simulink model "LDSNEmo_TestBench"  (R2020b)
settings: Solver=FixedStepAuto  StartTime=0.0  StopTime=1477  FixedStep=0.01  RelTol=1e-3
model workspace (MAT data in the model file):
  C_RR = 0.0103752252297
  SampleTime = 0.01
  StopTime = 1477
  UncertaintyRollerDynamometer = 0.796984855506
  VehMass = 929
  c_w = 0.37
  cycle : timeseries (value not decoded)
  i_gear = 5.6813
  p = 2.5
  power_map_LE = [81.3594367777 81.3594367777 88.9151238368 69.3920543425 121.856227925 33.5913037104 56.5214963128 60.6342218487 61.1595876762 53.4292335319 53.4133899816 35.6771556802 ... (16260 elements, 60x271)]
  power_map_Mot = [0 74.834999341 40.2428359465 95.3690451807 75.6091573236 114.707467852 143.074401876 144.922747771 177.284289075 184.351766643 192.404587732 197.413952644 ... (16260 elements, 60x271)]
  r_dyn = 0.275233869952
undefined symbols (not defined in the file): DiscIntNeverNeededParam, gravity, UncertaintyMappedLosses, UncertaintyTabledConsumption, v_HA
libraries: Constant_Environment x1, Driver_PI x1, Longitudinal_DrivingCycles x1, Acceleration_Calculation x1, Air_Resistance x1, Roll_Resistance x1, Slope_Resistance x1, Simple_Auxiliary x1, Electric_Drive_Tabled_Consumption x1, Gear_Stage x1, DCAC_Converter x1, Control_Unit_Simple x1
(part 2 of 3)

== system LDSNEmo_TestBench/Driver and Environment ==
  BUS_In : Inport
  BUS IN : Subsystem
      mask help:
      | <Author> Alexander Koch based on Stefan Müller, Stephan Rohr
      | <Date> 02/05/2017
      |
      | <Description>
      | Automated BUS IN Block for the Bus System. After the Bus In is connected and receives signals it is possible to choose the required signals by clicking on the block. After choosing the signals it is possible to push the Refresh button. This button builds the required amount of outputs, connects the Bus Selector and the Outputs and rename all the outputs with the corresponding signal name.
      |
      | The Block automaticlly disconnects the link to the library block after opening the first time
      |
      | <Parameters>
      | -
      |
      | <Inputs>
      | Bus [Bus]
      |
      | <Outputs>
      | Bus [Bus]
      | SignalName[-]
      mask init:
      | BusInInitFct()
      settings: OpenFcn=|
      | set_param(gcb(),'LinkStatus','none')
      | open_system(gcb(),'mask')
      | open_system(strcat(gcb(),'/Bus Selector'),'Parameter')
      mask DialogControl ParameterGroupVar Prompt: Refresh
      mask DialogControl RefreshOutputs Prompt: Refresh all Output Names
      mask DialogControl RefreshOutputs Callback: BusInInitFct()
  BUS OUT : Subsystem  mask{NumberofInputs=6, NameSys='Driver and Enironment'}
      mask prompts: NumberofInputs "Numper of costum inputs"; NameSys "Name of Bus Subsystem"
      mask help:
      | <Author> Alexander Koch based on Stefan Müller, Stephan Rohr
      | <Date> 02/05/2017
      |
      | <Description>
      | Automated BUS Out Block for the Bus System. Allows to enter the Number of costum inputs and the name of the bus system. After entering the parameters the required amout of Inputs are built and connected to the Bus Creator. The signal names that are connected to the inputs In1, ..., InN are automatically adopted at the Bus signal names and can be found in the Bus under the name of the Bus Subsystem. If the signal (line) to the Inport has no name, the name of the previous blocks outport is taken. If this is not possible, the name if the previous block is taken for the Bus signal name.
      |
      | Additional, there are two buttons. The Refresh Input Names refreshes all Input Names. This is required if signal names are changed or signals are connected for the first time. To build a new system or if another Subsystem is added between existing subsystems, the Refresh Bus Selector is required at every subsystem that is calculated after the new subsystem.
      |
      | The Block automaticlly disconnects the link to the library block after opening the first time
      |
      | <Parameters>
      | Number of costum inputs [-]
      | Name of Bus Subsystem ['abc']
      |
      | <Inputs>
      | Bus [Bus]
      | In1 [ ]
      |
      | <Outputs>
      | Bus [Bus]
      mask init:
      | BusRefreshInputs()
      settings: OpenFcn=|
      | set_param(gcb(),'LinkStatus','none')
      | open_system(gcb(),'mask')
      mask DialogControl Container3 Prompt: Refresh
      mask DialogControl RefreshInputNames Prompt: Refresh Input Names
      mask DialogControl RefreshInputNames Callback: BusRefreshLineNames()
      mask DialogControl RefreshBusSelector Prompt: Refresh Bus Selector
      mask DialogControl RefreshBusSelector Callback: BusRefreshBusSelector()
  Constant Environment : Constant_Environment/Constant Environment  Ground_Slope=0  Long_Wind_Speed=0  Ambient_P=101325  Ambient_Temp=293.15  LocalSampleTime=-1
  Driver PI : Driver_PI/Driver PI  ThrottleP=7  ThrottleI=1  BrakeP=7  BrakeI=1.5  WeightingFactorPrecontrol=0  MaxVehicleSpeed=80  hysteresis=0.05  LocalSampleTime=-1
  BUS_Out : Outport  VectorParamsAs1DForOutWhenUnconnected=off
  wires:
  BUS IN/1(BUS) -> BUS OUT/1(BUS)
  BUS OUT/1(BUS_OUT) -> BUS_Out/1
  BUS_In/1 -> BUS IN/1(BUS_In)
  BUS IN/2(v [m/s]) -> Driver PI/1
  Driver PI/1 -> BUS OUT/2(In1)
  Driver PI/2 -> BUS OUT/3(In2)
  Constant Environment/1 -> BUS OUT/4(In3)
  Constant Environment/2 -> BUS OUT/5(In4)
  BUS IN/3(VehSpd [m/s]) -> Driver PI/2
  Constant Environment/3 -> BUS OUT/6(In5)
  Constant Environment/4 -> BUS OUT/7(In6)

== system LDSNEmo_TestBench/Driving Cycle ==
  BUS_In : Inport
  BUS IN : Subsystem
      mask help:
      | <Author> Alexander Koch
      | <Date> 02/05/2017
      | <Predecessor> Stefan Müller, Stephan Rohr
      |
      | <Description>
      | Automated BUS IN Block for the Bus System. After the Bus In is connected and receives signals it is possible to choose the required signals by clicking on the block. After choosing the signals it is possible to push the Refresh button. This button builds the required amount of outputs, connects the Bus Selector and the Outputs and rename all the outputs with the corresponding signal name.
      |
      | The Block automaticlly disconnects the link to the library block after opening the first time
      |
      | <Parameters>
      | -
      |
      | <Inputs>
      | Bus [Bus]
      |
      | <Outputs>
      | Bus [Bus]
      | SignalName[-]
      mask init:
      | BusInInitFct()
      settings: OpenFcn=|
      | set_param(gcb(),'LinkStatus','none')
      | open_system(gcb(),'mask')
      | open_system(strcat(gcb(),'/Bus Selector'),'Parameter')
      mask DialogControl ParameterGroupVar Prompt: Refresh
      mask DialogControl RefreshOutputs Prompt: Refresh all Output Names
      mask DialogControl RefreshOutputs Callback: BusInInitFct()
  BUS OUT : Subsystem  mask{NumberofInputs=4, NameSys='DrivinCycle'}
      mask prompts: NumberofInputs "Numper of costum inputs"; NameSys "Name of Bus Subsystem"
      mask help:
      | <Author> Alexander Koch based on Stefan Müller, Stephan Rohr
      | <Date> 02/05/2017
      |
      | <Description>
      | Automated BUS Out Block for the Bus System. Allows to enter the Number of costum inputs and the name of the bus system. After entering the parameters the required amout of Inputs are built and connected to the Bus Creator. The signal names that are connected to the inputs In1, ..., InN are automatically adopted at the Bus signal names and can be found in the Bus under the name of the Bus Subsystem. If the signal (line) to the Inport has no name, the name of the previous blocks outport is taken. If this is not possible, the name if the previous block is taken for the Bus signal name.
      |
      | Additional, there are two buttons. The Refresh Input Names refreshes all Input Names. This is required if signal names are changed or signals are connected for the first time. To build a new system or if another Subsystem is added between existing subsystems, the Refresh Bus Selector is required at every subsystem that is calculated after the new subsystem.
      |
      | The Block automaticlly disconnects the link to the library block after opening the first time
      |
      | <Parameters>
      | Number of costum inputs [-]
      | Name of Bus Subsystem ['abc']
      |
      | <Inputs>
      | Bus [Bus]
      | In1 [ ]
      |
      | <Outputs>
      | Bus [Bus]
      mask init:
      | BusRefreshInputs()
      settings: OpenFcn=|
      | set_param(gcb(),'LinkStatus','none')
      | open_system(gcb(),'mask')
      mask DialogControl Container3 Prompt: Refresh
      mask DialogControl RefreshInputNames Prompt: Refresh Input Names
      mask DialogControl RefreshInputNames Callback: BusRefreshLineNames()
      mask DialogControl RefreshBusSelector Prompt: Refresh Bus Selector
      mask DialogControl RefreshBusSelector Callback: BusRefreshBusSelector()
  Longitudinal Driving Cycles : Longitudinal_DrivingCycles/Longitudinal Driving Cycles  dcname=Custom_Driving_Cycle  dccircuits=1  dc_speed=cycle  dc_gear=[]  LocalSampleTime=-1
  Terminator : Terminator
  BUS_Out : Outport  VectorParamsAs1DForOutWhenUnconnected=off
  wires:
  BUS IN/1(BUS) -> BUS OUT/1(BUS)
  BUS OUT/1(BUS_OUT) -> BUS_Out/1
  BUS_In/1 -> BUS IN/1(BUS_In)
  Longitudinal Driving Cycles/1 -> BUS OUT/2(In1)  "v [m/s]"
  Longitudinal Driving Cycles/2 -> BUS OUT/3(In2)
  Longitudinal Driving Cycles/3 -> BUS OUT/4(In3)
  Longitudinal Driving Cycles/4 -> BUS OUT/5(In4)
  BUS IN/2(VehSpd [m/s]) -> Terminator/1

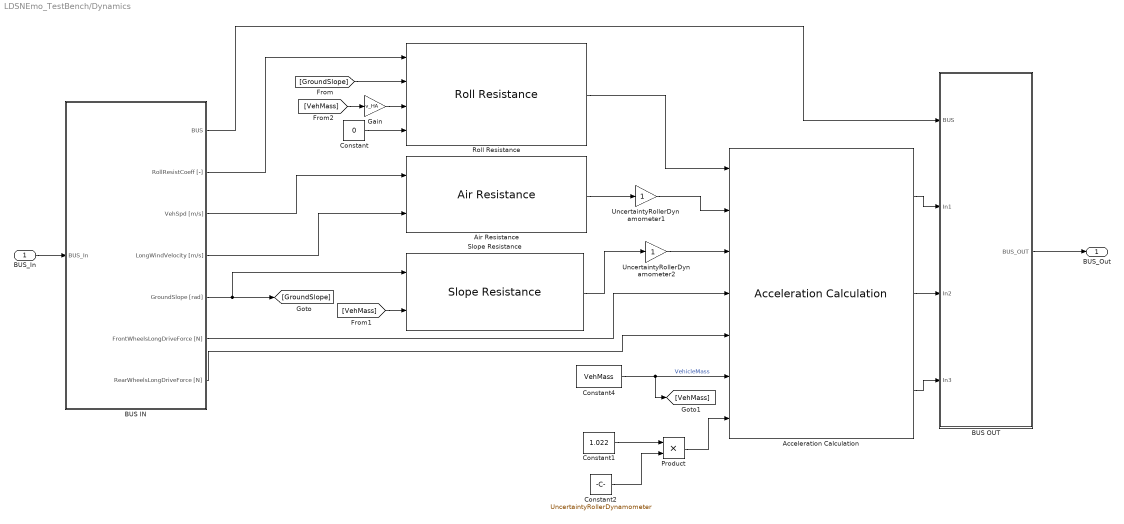
== system LDSNEmo_TestBench/Dynamics ==
  BUS_In : Inport
  Acceleration Calculation : Acceleration_Calculation/Acceleration Calculation  InitialCondition=0  LocalSampleTime=-1
  Air Resistance : Air_Resistance/Air Resistance  A_st=1.96  Roh_Air=rho_L  c_w=c_w  LocalSampleTime=-1
  BUS IN : Subsystem
      mask help:
      | <Author> Alexander Koch
      | <Date> 02/05/2017
      | <Predecessor> Stefan Müller, Stephan Rohr
      |
      | <Description>
      | Automated BUS IN Block for the Bus System. After the Bus In is connected and receives signals it is possible to choose the required signals by clicking on the block. After choosing the signals it is possible to push the Refresh button. This button builds the required amount of outputs, connects the Bus Selector and the Outputs and rename all the outputs with the corresponding signal name.
      |
      | The Block automaticlly disconnects the link to the library block after opening the first time
      |
      | <Parameters>
      | -
      |
      | <Inputs>
      | Bus [Bus]
      |
      | <Outputs>
      | Bus [Bus]
      | SignalName[-]
      mask init:
      | BusInInitFct()
      settings: OpenFcn=|
      | set_param(gcb(),'LinkStatus','none')
      | open_system(gcb(),'mask')
      | open_system(strcat(gcb(),'/Bus Selector'),'Parameter')
      mask DialogControl ParameterGroupVar Prompt: Refresh
      mask DialogControl RefreshOutputs Prompt: Refresh all Output Names
      mask DialogControl RefreshOutputs Callback: BusInInitFct()
  BUS OUT : Subsystem  mask{NumberofInputs=3, NameSys='Dynamics'}
      mask prompts: NumberofInputs "Numper of costum inputs"; NameSys "Name of Bus Subsystem"
      mask help:
      | <Author> Alexander Koch
      | <Date> 02/05/2017
      | <Predecessor> Stefan Müller, Stephan Rohr
      |
      | <Description>
      | Automated BUS Out Block for the Bus System. Allows to enter the Number of costum inputs and the name of the bus system. After entering the parameters the required amout of Inputs are built and connected to the Bus Creator. The signal names that are connected to the inputs In1, ..., InN are automatically adopted at the Bus signal names and can be found in the Bus under the name of the Bus Subsystem. If the signal (line) to the Inport has no name, the name of the previous blocks outport is taken. If this is not possible, the name if the previous block is taken for the Bus signal name.
      |
      | Additional, there are two buttons. The Refresh Input Names refreshes all Input Names. This is required if signal names are changed or signals are connected for the first time. To build a new system or if another Subsystem is added between existing subsystems, the Refresh Bus Selector is required at every subsystem that is calculated after the new subsystem.
      |
      | The Block automaticlly disconnects the link to the library block after opening the first time
      |
      | <Parameters>
      | Number of costum inputs [-]
      | Name of Bus Subsystem ['abc']
      |
      | <Inputs>
      | Bus [Bus]
      | In1 [ ]
      |
      | <Outputs>
      | Bus [Bus]
      mask init:
      | BusRefreshInputs()
      settings: OpenFcn=|
      | set_param(gcb(),'LinkStatus','none')
      | open_system(gcb(),'mask')
      mask DialogControl Container3 Prompt: Refresh
      mask DialogControl RefreshInputNames Prompt: Refresh Input Names
      mask DialogControl RefreshInputNames Callback: BusRefreshLineNames()
      mask DialogControl RefreshBusSelector Prompt: Refresh Bus Selector
      mask DialogControl RefreshBusSelector Callback: BusRefreshBusSelector()
  Constant : Constant  Value=0
  Constant1 : Constant  Value=1.022
  Constant2 : Constant  Value=UncertaintyRollerDynamometer
  Constant4 : Constant  Value=VehMass  SampleTime=-1
  Gain : Gain  Gain=v_HA
  Product : Product
  Roll Resistance : Roll_Resistance/Roll Resistance  Gravity=gravity  LocalSampleTime=-1
  Slope Resistance : Slope_Resistance/Slope Resistance  Gravity=gravity  LocalSampleTime=-1
  UncertaintyRollerDynamometer1 : Gain
  UncertaintyRollerDynamometer2 : Gain
  BUS_Out : Outport  VectorParamsAs1DForOutWhenUnconnected=off
  wires:
  BUS IN/1(BUS) -> BUS OUT/1(BUS)
  BUS OUT/1(BUS_OUT) -> BUS_Out/1
  BUS_In/1 -> BUS IN/1(BUS_In)
  BUS IN/2(RollResistCoeff [-]) -> Roll Resistance/1
  BUS IN/4(LongWindVelocity [m/s]) -> Air Resistance/2
  [GroundSlope] -> Roll Resistance/2
  BUS IN/5(GroundSlope [rad]) -> Slope Resistance/1, [GroundSlope]
  Air Resistance/1 -> UncertaintyRollerDynamometer1/1
  Slope Resistance/1 -> UncertaintyRollerDynamometer2/1
  BUS IN/6(FrontWheelsLongDriveForce [N]) -> Acceleration Calculation/4
  BUS IN/7(RearWheelsLongDriveForce [N]) -> Acceleration Calculation/5
  Constant4/1 -> [VehMass], Acceleration Calculation/6  "VehicleMass"
  [VehMass] -> Slope Resistance/2
  [VehMass] -> Gain/1
  Constant/1 -> Roll Resistance/4
  Constant1/1 -> Product/1
  Acceleration Calculation/1 -> BUS OUT/2(In1)
  Acceleration Calculation/2 -> BUS OUT/3(In2)
  Acceleration Calculation/3 -> BUS OUT/4(In3)
  BUS IN/3(VehSpd [m/s]) -> Air Resistance/1
  Roll Resistance/1 -> Acceleration Calculation/1
  UncertaintyRollerDynamometer1/1 -> Acceleration Calculation/2
  UncertaintyRollerDynamometer2/1 -> Acceleration Calculation/3
  Gain/1 -> Roll Resistance/3
  Product/1 -> Acceleration Calculation/7
  Constant2/1 -> Product/2

== system LDSNEmo_TestBench/Power Source ==
  note: During the experiments the vehicle Smart Fortwo
      | was pluged in to a battery simulator, which provides
      | a power source with constant voltage.
  BUS_In : Inport
  Add : Sum
  BUS IN : Subsystem
      mask help:
      | <Author> Alexander Koch based on Stefan Müller, Stephan Rohr
      | <Date> 02/05/2017
      |
      | <Description>
      | Automated BUS IN Block for the Bus System. After the Bus In is connected and receives signals it is possible to choose the required signals by clicking on the block. After choosing the signals it is possible to push the Refresh button. This button builds the required amount of outputs, connects the Bus Selector and the Outputs and rename all the outputs with the corresponding signal name.
      |
      | The Block automaticlly disconnects the link to the library block after opening the first time
      |
      | <Parameters>
      | -
      |
      | <Inputs>
      | Bus [Bus]
      |
      | <Outputs>
      | Bus [Bus]
      | SignalName[-]
      mask init:
      | BusInInitFct()
      settings: OpenFcn=|
      | set_param(gcb(),'LinkStatus','none')
      | open_system(gcb(),'mask')
      | open_system(strcat(gcb(),'/Bus Selector'),'Parameter')
      mask DialogControl ParameterGroupVar Prompt: Refresh
      mask DialogControl RefreshOutputs Prompt: Refresh all Output Names
      mask DialogControl RefreshOutputs Callback: BusInInitFct()
  BUS OUT : Subsystem  mask{NumberofInputs=3, NameSys='Powersource'}
      mask prompts: NumberofInputs "Numper of costum inputs"; NameSys "Name of Bus Subsystem"
      mask help:
      | <Author> Alexander Koch based on Stefan Müller, Stephan Rohr
      | <Date> 02/05/2017
      |
      | <Description>
      | Automated BUS Out Block for the Bus System. Allows to enter the Number of costum inputs and the name of the bus system. After entering the parameters the required amout of Inputs are built and connected to the Bus Creator. The signal names that are connected to the inputs In1, ..., InN are automatically adopted at the Bus signal names and can be found in the Bus under the name of the Bus Subsystem. If the signal (line) to the Inport has no name, the name of the previous blocks outport is taken. If this is not possible, the name if the previous block is taken for the Bus signal name.
      |
      | Additional, there are two buttons. The Refresh Input Names refreshes all Input Names. This is required if signal names are changed or signals are connected for the first time. To build a new system or if another Subsystem is added between existing subsystems, the Refresh Bus Selector is required at every subsystem that is calculated after the new subsystem.
      |
      | The Block automaticlly disconnects the link to the library block after opening the first time
      |
      | <Parameters>
      | Number of costum inputs [-]
      | Name of Bus Subsystem ['abc']
      |
      | <Inputs>
      | Bus [Bus]
      | In1 [ ]
      |
      | <Outputs>
      | Bus [Bus]
      mask init:
      | BusRefreshInputs()
      settings: OpenFcn=|
      | set_param(gcb(),'LinkStatus','none')
      | open_system(gcb(),'mask')
      mask DialogControl Container3 Prompt: Refresh
      mask DialogControl RefreshInputNames Prompt: Refresh Input Names
      mask DialogControl RefreshInputNames Callback: BusRefreshLineNames()
      mask DialogControl RefreshBusSelector Prompt: Refresh Bus Selector
      mask DialogControl RefreshBusSelector Callback: BusRefreshBusSelector()
  Constant Power Source : Subsystem  mask(SB){MaxPower=400000, MinPower=-10000}
      mask prompts: MaxPower "Maximum Power [W]"; MinPower "Minimum Power [W]"
      mask help:
      | <Author> Tony Weiss based on Nikolaos Wassiliadis, Michael Baumann </Author>
      | <Date> 22/04/2018 </Date>
      |
      | <Description>
      | Inside this battery model is the battery cell Panasonic 18650PF which calculates all cell parameters. Through the number of cells parallel and serial, the battery power and voltage is calculated. The model therefore needs the initals values of SOC, U_RC1 and U_RC2 of the cell.
      | </Description>
      mask Help:
      | <Parameters>
      | Cells Serial [-]
      | 	<Min> 1 </Min>
      | Cells Parallel [-]
      | 	<Min> 1 </Min>
      | Initial Cell State [3x1]
      | 	--> [SOC;U_RC1;U_RC2]
      | 
      | 	SOC: 	<Min> 0 </Min>
      | 		<Max> 1 </Max>
      | 	U_RC1:	<Min> 0 </Min>
      | 	U_RC2:	<Min> 0 </Min>
      | </Parameters>
      | 
      | <Inputs>
      | CellPara_x_k [-]
      | 	3x1 Vector --> [SOC;U_RC1;U_RC2]
      | CellVoltage_x_k [V]
      | BatPowerReq [W]
      | 	<sign orientation> [+] discharge </sign orientation>
      | </Inputs>
      | 
      | <Outputs>
      | SOC [-]
      | 	<Min> 0 </Min>
      | 	<Max> 1 </Max>
      | CellPara_x_k+1 [-]
      | 	3x1 Vector --> [SOC;U_RC1;U_RC2]
      | CellVoltage_x_k+1 [V]
      | BatPowerAvl [W]
      | 	<sign orientation> [+] discharge </sign orientation>
      | </Outputs>
      mask DialogControl Container3 Prompt: Documentation:
      mask DialogControl Control2 Prompt: %<MaskHelp>
  Simple Auxiliary : Simple_Auxiliary/Simple Auxiliary  AuxPower=114.6055  LocalSampleTime=0
  BUS_Out : Outport  VectorParamsAs1DForOutWhenUnconnected=off
  wires:
  BUS IN/1(BUS) -> BUS OUT/1(BUS)
  BUS OUT/1(BUS_OUT) -> BUS_Out/1
  BUS_In/1 -> BUS IN/1(BUS_In)
  Constant Power Source/1(ActualPower [W]) -> BUS OUT/2(In1)
  Constant Power Source/2(MaxPower [W]) -> BUS OUT/3(In2)
  Constant Power Source/3(MinPower [W]) -> BUS OUT/4(In3)
  BUS IN/2(PowertrainPowerReq [W]) -> Add/2
  Add/1 -> Constant Power Source/1(RequiredPower [W])
  Simple Auxiliary/1 -> Add/1  "AuxiliariesPower [W]"

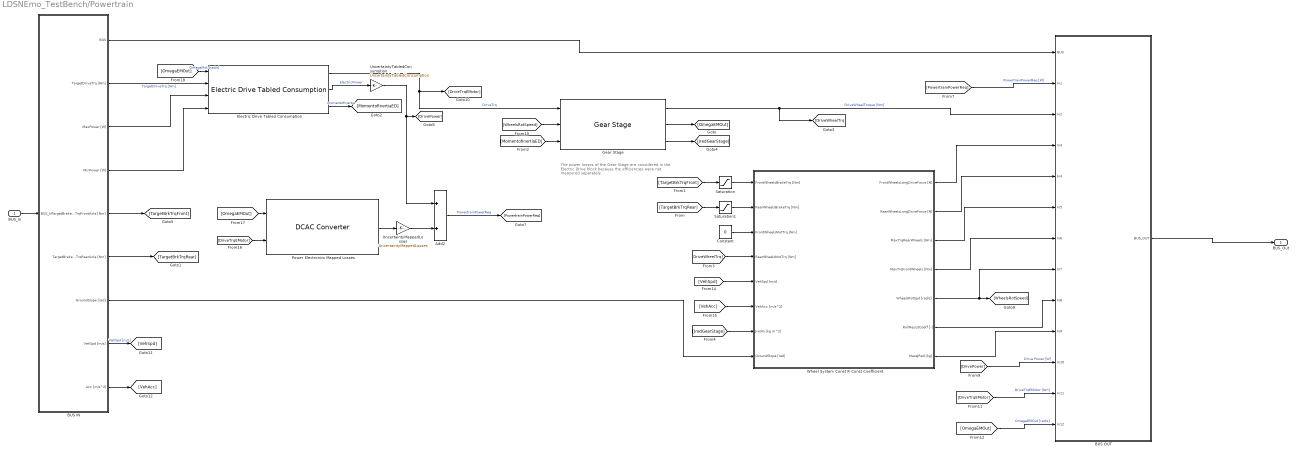
== system LDSNEmo_TestBench/Powertrain ==
  note: The power losses of the Gear Stage are considered
      | in the Electric Drive block because the efficiencies were
      | not measured separately.
  BUS_In : Inport
  Add2 : Sum
  BUS IN : Subsystem
      mask help:
      | <Author> Alexander Koch based on Stefan Müller, Stephan Rohr
      | <Date> 02/05/2017
      |
      | <Description>
      | Automated BUS IN Block for the Bus System. After the Bus In is connected and receives signals it is possible to choose the required signals by clicking on the block. After choosing the signals it is possible to push the Refresh button. This button builds the required amount of outputs, connects the Bus Selector and the Outputs and rename all the outputs with the corresponding signal name.
      |
      | The Block automaticlly disconnects the link to the library block after opening the first time
      |
      | <Parameters>
      | -
      |
      | <Inputs>
      | Bus [Bus]
      |
      | <Outputs>
      | Bus [Bus]
      | SignalName[-]
      mask init:
      | BusInInitFct()
      settings: OpenFcn=|
      | set_param(gcb(),'LinkStatus','none')
      | open_system(gcb(),'mask')
      | open_system(strcat(gcb(),'/Bus Selector'),'Parameter')
      mask DialogControl ParameterGroupVar Prompt: Refresh
      mask DialogControl RefreshOutputs Prompt: Refresh all Output Names
      mask DialogControl RefreshOutputs Callback: BusInInitFct()
  BUS OUT : Subsystem  mask{NumberofInputs=12, NameSys='Powertrain'}
      mask prompts: NumberofInputs "Numper of costum inputs"; NameSys "Name of Bus Subsystem"
      mask help:
      | <Author> Alexander Koch based on Stefan Müller, Stephan Rohr
      | <Date> 02/05/2017
      |
      | <Description>
      | Automated BUS Out Block for the Bus System. Allows to enter the Number of costum inputs and the name of the bus system. After entering the parameters the required amout of Inputs are built and connected to the Bus Creator. The signal names that are connected to the inputs In1, ..., InN are automatically adopted at the Bus signal names and can be found in the Bus under the name of the Bus Subsystem. If the signal (line) to the Inport has no name, the name of the previous blocks outport is taken. If this is not possible, the name if the previous block is taken for the Bus signal name.
      |
      | Additional, there are two buttons. The Refresh Input Names refreshes all Input Names. This is required if signal names are changed or signals are connected for the first time. To build a new system or if another Subsystem is added between existing subsystems, the Refresh Bus Selector is required at every subsystem that is calculated after the new subsystem.
      |
      | The Block automaticlly disconnects the link to the library block after opening the first time
      |
      | <Parameters>
      | Number of costum inputs [-]
      | Name of Bus Subsystem ['abc']
      |
      | <Inputs>
      | Bus [Bus]
      | In1 [ ]
      |
      | <Outputs>
      | Bus [Bus]
      mask init:
      | BusRefreshInputs()
      settings: OpenFcn=|
      | set_param(gcb(),'LinkStatus','none')
      | open_system(gcb(),'mask')
      mask DialogControl Container3 Prompt: Refresh
      mask DialogControl RefreshInputNames Prompt: Refresh Input Names
      mask DialogControl RefreshInputNames Callback: BusRefreshLineNames()
      mask DialogControl RefreshBusSelector Prompt: Refresh Bus Selector
      mask DialogControl RefreshBusSelector Callback: BusRefreshBusSelector()
  Constant : Constant  Value=0
  Electric Drive Tabled Consumption : Electric_Drive_Tabled_Consumption/Electric Drive Tabled Consumption  inertia=0.03  mass=1  OM_M_Pel_Map=power_map_Mot  M_MotVector=torque_Mot  OM_MotVector=omega_Mot  M_Full_Load=[128 128 128 127 127 126 126 126 126 124 119 114 109 103 100 94 89 85 79 75 70 68 67 65 63 62 60 58 59 60 62 63 63 62 61 60 58 57 55 53 51 50 48 46 45 43 42 40 39 38 36 35 34 32 31 30 29 28 26 25 24]  OM_Full_Load=[0 11.4144533080429 22.8289066160858 34.2433599241288 45.6578132321717 57.1769862953342 68.5914396033771 80.0058929114201 91.4203462194630 102.834799527506 114.249252835549 125.663706143592 137.078159451635 148.492612759678 160.011785822840 171.426239130883 182.840692438926 194.255145746969 205.669599055012 217.084052363055 228.498505671098 239.912958979141 251.327412287183 262.846585350346 274.261038658389 285.675491966432 297.089945274475 308.504398582518 319.918851890561 331.333305198604 342.747758506646 354.162211814689 365.681384877852 377.095838185895 388.510291493938 399.924744801981 411.339198110024 422.753651418066 434.168104726109 445.582558034152 456.997011342195 468.516184405358 479.930637713401 491.345091021444 502.759544329487 514.173997637529 525.588450945572 537.002904253615 548.417357561658 559.831810869701 571.350983932864 582.765437240907 594.179890548950 605.594343856992 617.008797165035 628.423250473078 639.837703781121 651.252157089164 662.666610397207 674.185783460370 685.600236768413]  M_Min_Load=[0 0 0 0 0 0 0 0 0 0 0 0 0 0 0 0 0 0 0 0 0 0 0 0 0 0 0 0 0 0 0 0 0 0 0 0 0 0 0 0 0 0 0 0 0 0 0 0 0 0 0 0 0 0 0 0 0 0 0 0 0]  OM_Min_Load=[0 11.4144533080429 22.8289066160858 34.2433599241288 45.6578132321717 57.1769862953342 68.5914396033771 80.0058929114201 91.4203462194630 102.834799527506 114.249252835549 125.663706143592 137.078159451635 148.492612759678 160.011785822840 171.426239130883 182.840692438926 194.255145746969 205.669599055012 217.084052363055 228.498505671098 239.912958979141 251.327412287183 262.846585350346 274.261038658389 285.675491966432 297.089945274475 308.504398582518 319.918851890561 331.333305198604 342.747758506646 354.162211814689 365.681384877852 377.095838185895 388.510291493938 399.924744801981 411.339198110024 422.753651418066 434.168104726109 445.582558034152 456.997011342195 468.516184405358 479.930637713401 491.345091021444 502.759544329487 514.173997637529 525.588450945572 537.002904253615 548.417357561658 559.831810869701 571.350983932864 582.765437240907 594.179890548950 605.594343856992 617.008797165035 628.423250473078 639.837703781121 651.252157089164 662.666610397207 674.185783460370 685.600236768413]  LocalSampleTime=-1
  Gear Stage : Gear_Stage/Gear Stage  iGear=i_gear  eta=1  JredGetr=0.19  LocalSampleTime=-1
  Power Electronics Mapped Losses : DCAC_Converter/DCAC Converter  W_Vektor=omega_LE  M_Vektor_motgen=torque_LE  P_Loss=power_map_LE  LocalSampleTime=-1
  Saturation : Saturate  UpperLimit=0  LowerLimit=-inf
  Saturation1 : Saturate  UpperLimit=0  LowerLimit=-inf
  UncertaintyMappedLosses : Gain  Gain=UncertaintyMappedLosses
  UncertaintyTabledConsumption : Gain  Gain=UncertaintyTabledConsumption
  Wheel System Const R Const Coefficient : Subsystem  mask(SB){Wheel_Radius=r_dyn, Wheel_Roll_Resistance=C_RR, Wheel_Roll_Resistance_Dyn=0, mu_Tyre=0.7, J_FourWheels=4, Gravity=gravity, Wheelbase=1.863, COG_Height=0.5, COG_Front=1.1178, COG_Rear=0.7452, Veh_Mass=VehMass, LocalSampleTime=-1}
      mask prompts: Wheel_Radius "Wheel Radius [m]"; Wheel_Roll_Resistance "Roll Resistance Coefficient [-]"; Wheel_Roll_Resistance_Dyn "Dynamic Roll Resistance Coefficient [s/m]"; mu_Tyre "Friction Coefficient between Wheel/Road [-]"; J_FourWheels "Inertia Moment of four Wheels [kg m^2]"; Gravity "Gravity [m/s^2]"; Wheelbase "Wheelbase [m]"; COG_Height "Height Center of Gravity over Ground [m]"; COG_Front "Distance from Center of Gravity to Front Axle [m]"; COG_Rear "Distance from Center of Gravity to Rear Axle [m]"; Veh_Mass "Vehicle Mass [kg]"; LocalSampleTime "Local System Sample-Time [s]"
      mask help:
      | <Author> Alexander Koch, Benedikt Danquah based on Stefan Müller [1], Stephan Rohr [2]  </Author>
      | <Date> 15/01/2018 </Date>
      | <Sources>
      | [1] S. Mueller, S. Rohr, und et al, Hrsg, Analysing the Influence of Driver Behaviour and Tuning Measures on Battery Aging and Residual Value of Electric Vehicles, 2017
      | </Sources>
      |
      | <Description>
      | Calculates the longitudinal forces of the front and rear wheels, the rotational speed of the wheels and gives the roll resistant coefficient as an output. There are two roll resistant coefficients. A static parameter and a dynamic one. The dynamic roll resistant coefficient is mutliplied with the velocity and added to the static coefficient. Slip can not be represented. The moment of inertia is transfered to a mass.
      | </Description>
      mask init:
      | GlobalSampleTime = CalcGlobalSampleTime(LocalSampleTime);
      mask Help:
      | <Parameters>
      | Wheel Radius [m]
      | 	<Min> >0 </Min>
      | Roll Resistance Coefficient [-]
      | 	<Min> 0 </Min>
      | Dynamic Roll Resistance Coefficient [s/m]
      | Friction Coefficient between Wheel/Road [-]
      | Inertia Moment of four Wheels [kg m^2]
      | Gravity [m/s^2]
      | Wheelbase [m]
      | Height Center of Gravity over Ground [m]
      | Distance from Center of Gravity to Front Axle [m]
      | Distance from Center of Gravity to Rear Axle [m]
      | Local System Sample-Time [s]
      | 	<Min> GlobalSampleTime </Min>
      | Global Sample-Time [s]
      | </Parameters>
      | 
      | <Inputs>
      | FrontWheelsBrakeTrq [Nm]
      | 	 <sign orientation> [-] results in negative longitudinal driving Force </sign orientation>
      | RearWheelsBrakeTrq [Nm]
      | 	<sign orientation> [-] results in negative longitudinal driving Force </sign orientation>
      | FrontWheelsMotTrq [Nm]
      | 	<sign orientation> [+] results in positive longitudinal driving force </sign orientation>
      | RearWheelsMotTrq [Nm]
      | 	<sign orientation> [+] results in positive longitudinal driving force </sign orientation>
      | VehSpd [m/s]
      | VehAcc [m/s^2]
      | JRedIn [kg m^2]
      | GroundSlope [rad]
      | MassVehicle [kg]
      | </Inputs>
      | 
      | <Outputs>
      | FrontWheelsLongDriveForce [N]
      | RearWheelsLonDriveForce [N]
      | MaxTrqFrontWheels [Nm]
      | MaxTrqRearWheels [Nm]
      | WheelsRotSpd [rad/s]
      | RollResistCoeff [-]
      | MassJRed [kg]
      | </Outputs>
      | <Sources>
      | [1] S. Mueller, S. Rohr, W. Schmid, and M. Lienkamp, “Analysing the Influence of Driver Behaviour and Tuning Measures on Battery Aging and Residual Value of Electric Vehicles,” in Proc. EVS30 Symposium, Stuttgart, 2017, pp. 1–12.
      | [2] S. Rohr, “Technisch-wirtschaftliche Analyse des Zweitnutzungs- potentials von Lithium-Ionen-Traktionsbatterien,” Dissertation, Institute of Automotive Technology, Technical University Munich, Munich, 2018.
      | </Sources>
      mask TypeOptions Wheel_Radius: Wheel_Radius/Value
      mask TypeOptions Wheel_Roll_Resistance: Wheel_Roll_Resistance_Coeff/Value
      mask TypeOptions Wheel_Roll_Resistance_Dyn: Wheel_Roll_Resistance_Coeff_Dyn/Value
      mask TypeOptions mu_Tyre: mu_tyre/Value
      mask TypeOptions J_FourWheels: J_FourWheels/Value
      mask TypeOptions Gravity: Gravity/Value
      mask TypeOptions Wheelbase: Wheelbase/Value
      mask TypeOptions COG_Height: COG_Height/Value
      mask TypeOptions COG_Front: COG_Front/Value
      mask TypeOptions COG_Rear: COG_Rear/Value
      mask TypeOptions Veh_Mass: Vehicle_Mass/Value
      mask TypeOptions LocalSampleTime: FrontWheelsBrakeTrq [Nm]/SampleTime | RearWheelsBrakeTrq [Nm]/SampleTime | FrontWheelsMotTrq [Nm]/SampleTime | RearWheelsMotTrq [Nm]/SampleTime | VehSpd [m//s]/SampleTime | VehAcc [m//s^2]/SampleTime | JredIn [kg m^2]/SampleTime | GroundSlope [rad]/SampleTime
      mask DialogControl Container3 Prompt: Documentation
      mask DialogControl Control2 Prompt: %<MaskHelp>
      mask DialogControl Container5 Prompt: Sample Time
      mask Display:
      | [picturexpos,pictureypos,picturewidth,pictureheight] = ...
      |     CalcBlockPicturePosition(gcb,1,0.01,0.1,120,120); % calculating picture position depending on Block size and minimum margin size
      | image('Wheel_System_Const_R.svg',[picturexpos pictureypos picturewidth pictureheight]); % plot picture to block
  BUS_Out : Outport  VectorParamsAs1DForOutWhenUnconnected=off
  wires:
  BUS IN/1(BUS) -> BUS OUT/1(BUS)
  BUS_In/1 -> BUS IN/1(BUS_In)
  [TargetBrkTrqFront] -> Saturation/1
  [TargetBrkTrqRear] -> Saturation1/1
  BUS IN/5(TargetBrakeTrqFrontAxle [Nm]) -> [TargetBrkTrqFront]
  BUS IN/2(TargetDriveTrq [Nm]) -> Electric Drive Tabled Consumption/2  "TargetDriveTrq [Nm]"
  Electric Drive Tabled Consumption/1 -> Gear Stage/1, [DriveTrqEMotor]  "DriveTrq"
  Gear Stage/2 -> [OmegaEMOut]
  Constant/1 -> Wheel System Const R Const Coefficient/3(FrontWheelsMotTrq [Nm])
  [MomentofInertiaED] -> Gear Stage/3
  Gear Stage/1 -> [DriveWheelTrq], BUS OUT/3(In2)  "DriveWheelTorque [Nm]"
  [DriveWheelTrq] -> Wheel System Const R Const Coefficient/4(RearWheelsMotTrq [Nm])
  Gear Stage/3 -> [JredGearStage]
  [JredGearStage] -> Wheel System Const R Const Coefficient/7(JredIn [kg m^2])
  Wheel System Const R Const Coefficient/1(FrontWheelsLongDriveForce [N]) -> BUS OUT/4(In3)
  Wheel System Const R Const Coefficient/2(RearWheelsLongDriveForce [N]) -> BUS OUT/5(In4)
  Wheel System Const R Const Coefficient/3(MaxTrqRearWheels [Nm]) -> BUS OUT/6(In5)
  Wheel System Const R Const Coefficient/4(MaxTrqFrontWheels [Nm]) -> BUS OUT/7(In6)
  Wheel System Const R Const Coefficient/5(WheelsRotSpd [rad/s]) -> [WheelsRotSpeed], BUS OUT/8(In7)
  Wheel System Const R Const Coefficient/6(RollResistCoeff [-]) -> BUS OUT/9(In8)
  Wheel System Const R Const Coefficient/7(MassJRed [kg]) -> BUS OUT/10(In9)
  Electric Drive Tabled Consumption/2 -> UncertaintyTabledConsumption/1  "ElectricPower"
  Add2/1 -> [PowertrainPowerReq]  "PowertrainPowerReq"
  BUS IN/7(GroundSlope [rad]) -> Wheel System Const R Const Coefficient/8(GroundSlope [rad])
  Saturation/1 -> Wheel System Const R Const Coefficient/1(FrontWheelsBrakeTrq [Nm])
  Saturation1/1 -> Wheel System Const R Const Coefficient/2(RearWheelsBrakeTrq [Nm])
  [PowertrainPowerReq] -> BUS OUT/2(In1)  "PowertrainPowerReq [W]"
  [DrivePower] -> BUS OUT/11(In10)  "Drive Power [W]"
  [WheelsRotSpeed] -> Gear Stage/2
  [DriveTrqEMotor] -> BUS OUT/12(In11)  "DriveTrqEMotor [Nm]"
  [OmegaEMOut] -> BUS OUT/13(In12)  "OmegaEMOut [rad/s]"
  BUS IN/6(TargetBrakeTrqRearAxle [Nm]) -> [TargetBrkTrqRear]
  BUS IN/8(VehSpd [m/s]) -> [VehSpd]  "VehSpd [m/s]"
  [VehSpd] -> Wheel System Const R Const Coefficient/5(VehSpd [m/s])
  BUS IN/9(Acc [m/s^2]) -> [VehAcc]
  [VehAcc] -> Wheel System Const R Const Coefficient/6(VehAcc [m/s^2])
  [DriveTrqEMotor] -> Power Electronics Mapped Losses/2
  [OmegaEMOut] -> Power Electronics Mapped Losses/1
  Power Electronics Mapped Losses/1 -> UncertaintyMappedLosses/1
  [OmegaEMOut] -> Electric Drive Tabled Consumption/1  "OmegaMot [rad/s]"
  Electric Drive Tabled Consumption/3 -> [MomentofInertiaED]  "momentofinertia"
  BUS IN/3(MaxPower [W]) -> Electric Drive Tabled Consumption/3
  BUS IN/4(MinPower [W]) -> Electric Drive Tabled Consumption/4
  BUS OUT/1(BUS_OUT) -> BUS_Out/1
  UncertaintyTabledConsumption/1 -> Add2/1, [DrivePower]
  UncertaintyMappedLosses/1 -> Add2/2

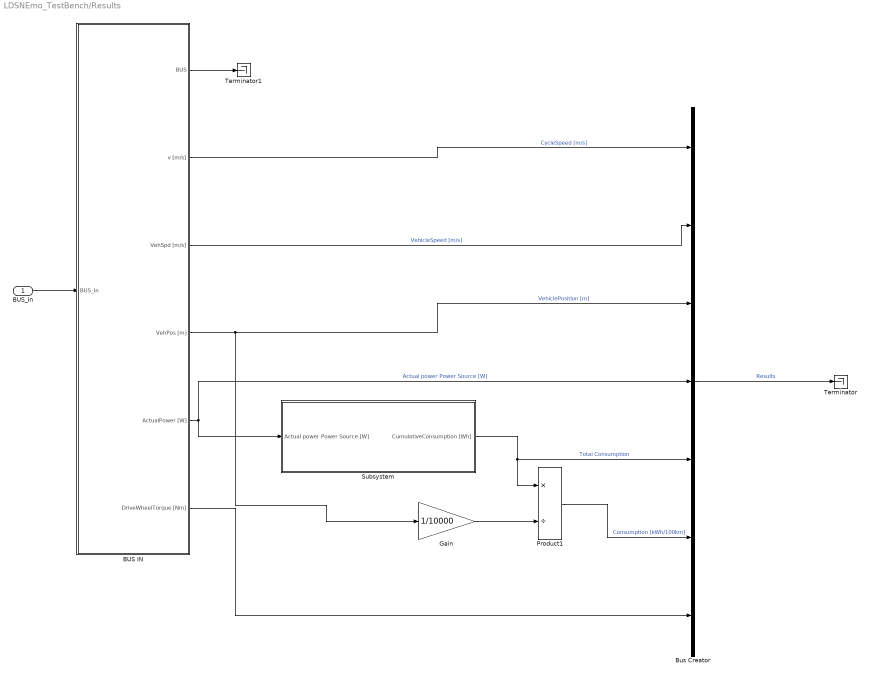
== system LDSNEmo_TestBench/Results ==
  BUS_In : Inport
  BUS IN : Subsystem
      mask help:
      | <Author> Alexander Koch
      | <Date> 02/05/2017
      | <Predecessor> Stefan Müller, Stephan Rohr
      |
      | <Description>
      | Automated BUS IN Block for the Bus System. After the Bus In is connected and receives signals it is possible to choose the required signals by clicking on the block. After choosing the signals it is possible to push the Refresh button. This button builds the required amount of outputs, connects the Bus Selector and the Outputs and rename all the outputs with the corresponding signal name.
      |
      | The Block automaticlly disconnects the link to the library block after opening the first time
      |
      | <Parameters>
      | -
      |
      | <Inputs>
      | Bus [Bus]
      |
      | <Outputs>
      | Bus [Bus]
      | SignalName[-]
      mask init:
      | BusInInitFct()
      settings: OpenFcn=|
      | set_param(gcb(),'LinkStatus','none')
      | open_system(gcb(),'mask')
      | open_system(strcat(gcb(),'/Bus Selector'),'Parameter')
      mask DialogControl ParameterGroupVar Prompt: Refresh
      mask DialogControl RefreshOutputs Prompt: Refresh all Output Names
      mask DialogControl RefreshOutputs Callback: BusInInitFct()
  Bus Creator : BusCreator  Inputs=7
  Gain : Gain  Gain=1/10000
  Product1 : Product  Inputs=*/
  Subsystem : Subsystem
  Terminator : Terminator
  Terminator1 : Terminator
  wires:
  BUS_In/1 -> BUS IN/1(BUS_In)
  BUS IN/1(BUS) -> Terminator1/1
  Bus Creator/1 -> Terminator/1  "Results"
  BUS IN/5(ActualPower [W]) -> Bus Creator/4, Subsystem/1(Actual power Power Source [W])  "Actual power Power Source [W]"
  BUS IN/2(v [m/s]) -> Bus Creator/1  "CycleSpeed [m/s]"
  BUS IN/3(VehSpd [m/s]) -> Bus Creator/2  "VehicleSpeed [m/s]"
  BUS IN/4(VehPos [m]) -> Bus Creator/3, Gain/1  "VehiclePosition [m]"
  BUS IN/6(DriveWheelTorque [Nm]) -> Bus Creator/7
  Gain/1 -> Product1/2
  Product1/1 -> Bus Creator/6  "Consumption [kWh/100km]"
  Subsystem/1(CumulativeConsumption [Wh]) -> Bus Creator/5, Product1/1  "Total Consumption"

== system LDSNEmo_TestBench/Timer and Bus Reset ==
  BUS_In : Inport
  Bus Creator : BusCreator  Inputs=1
  Bus Selector : BusSelector  OutputSignals=Dynamics,Powertrain,Powersource,VehicleControlUnit,Driver and Enironment,DrivinCycle  OutputAsBus=on
  Unit Delay : UnitDelay  SampleTime=-1  HasFrameUpgradeWarning=on
  BUS_Out : Outport  VectorParamsAs1DForOutWhenUnconnected=off
  wires:
  Bus Creator/1 -> BUS_Out/1
  Bus Selector/1 -> Unit Delay/1
  Unit Delay/1 -> Bus Creator/1  "Bus_Old"
  BUS_In/1 -> Bus Selector/1

== system LDSNEmo_TestBench/Vehicle Control Unit ==
  BUS_In : Inport
  BUS IN : Subsystem
      mask help:
      | <Author> Alexander Koch based on Stefan Müller, Stephan Rohr
      | <Date> 02/05/2017
      |
      | <Description>
      | Automated BUS IN Block for the Bus System. After the Bus In is connected and receives signals it is possible to choose the required signals by clicking on the block. After choosing the signals it is possible to push the Refresh button. This button builds the required amount of outputs, connects the Bus Selector and the Outputs and rename all the outputs with the corresponding signal name.
      |
      | The Block automaticlly disconnects the link to the library block after opening the first time
      |
      | <Parameters>
      | -
      |
      | <Inputs>
      | Bus [Bus]
      |
      | <Outputs>
      | Bus [Bus]
      | SignalName[-]
      mask init:
      | BusInInitFct()
      settings: OpenFcn=|
      | set_param(gcb(),'LinkStatus','none')
      | open_system(gcb(),'mask')
      | open_system(strcat(gcb(),'/Bus Selector'),'Parameter')
      mask DialogControl ParameterGroupVar Prompt: Refresh
      mask DialogControl RefreshOutputs Prompt: Refresh all Output Names
      mask DialogControl RefreshOutputs Callback: BusInInitFct()
  BUS OUT : Subsystem  mask{NumberofInputs=3, NameSys='VehicleControlUnit'}
      mask prompts: NumberofInputs "Numper of costum inputs"; NameSys "Name of Bus Subsystem"
      mask help:
      | <Author> Alexander Koch based on Stefan Müller, Stephan Rohr
      | <Date> 02/05/2017
      |
      | <Description>
      | Automated BUS Out Block for the Bus System. Allows to enter the Number of costum inputs and the name of the bus system. After entering the parameters the required amout of Inputs are built and connected to the Bus Creator. The signal names that are connected to the inputs In1, ..., InN are automatically adopted at the Bus signal names and can be found in the Bus under the name of the Bus Subsystem. If the signal (line) to the Inport has no name, the name of the previous blocks outport is taken. If this is not possible, the name if the previous block is taken for the Bus signal name.
      |
      | Additional, there are two buttons. The Refresh Input Names refreshes all Input Names. This is required if signal names are changed or signals are connected for the first time. To build a new system or if another Subsystem is added between existing subsystems, the Refresh Bus Selector is required at every subsystem that is calculated after the new subsystem.
      |
      | The Block automaticlly disconnects the link to the library block after opening the first time
      |
      | <Parameters>
      | Number of costum inputs [-]
      | Name of Bus Subsystem ['abc']
      |
      | <Inputs>
      | Bus [Bus]
      | In1 [ ]
      |
      | <Outputs>
      | Bus [Bus]
      mask init:
      | BusRefreshInputs()
      settings: OpenFcn=|
      | set_param(gcb(),'LinkStatus','none')
      | open_system(gcb(),'mask')
      mask DialogControl Container3 Prompt: Refresh
      mask DialogControl RefreshInputNames Prompt: Refresh Input Names
      mask DialogControl RefreshInputNames Callback: BusRefreshLineNames()
      mask DialogControl RefreshBusSelector Prompt: Refresh Bus Selector
      mask DialogControl RefreshBusSelector Callback: BusRefreshBusSelector()
  Control Unit Simple : Control_Unit_Simple/Control Unit Simple  Brake_Distribution_Front=0.7  MaxBrkTrq=448  MaxMotorTrq=110  LocalSampleTime=-1
  BUS_Out : Outport  VectorParamsAs1DForOutWhenUnconnected=off
  wires:
  BUS IN/1(BUS) -> BUS OUT/1(BUS)
  BUS OUT/1(BUS_OUT) -> BUS_Out/1
  BUS_In/1 -> BUS IN/1(BUS_In)
  Control Unit Simple/2 -> BUS OUT/3(In2)
  Control Unit Simple/3 -> BUS OUT/4(In3)
  Control Unit Simple/1 -> BUS OUT/2(In1)
  BUS IN/2(AccPedalPos [-]) -> Control Unit Simple/1
  BUS IN/3(BrakePedalPos [-]) -> Control Unit Simple/2

== system LDSNEmo_TestBench/Driver and Environment/BUS IN ==
  BUS_In : Inport
  Bus Selector : BusSelector  OutputSignals=DrivinCycle.v [m/s],Bus_Old.Dynamics.VehSpd [m/s]
  BUS : Outport  VectorParamsAs1DForOutWhenUnconnected=off
  v [m/s] : Outport  Port=2  VectorParamsAs1DForOutWhenUnconnected=off
  VehSpd [m/s] : Outport  Port=3  VectorParamsAs1DForOutWhenUnconnected=off
  wires:
  BUS_In/1 -> Bus Selector/1, BUS/1
  Bus Selector/1 -> v [m/s]/1  "<v [m/s]>"
  Bus Selector/2 -> VehSpd [m/s]/1  "<VehSpd [m/s]>"

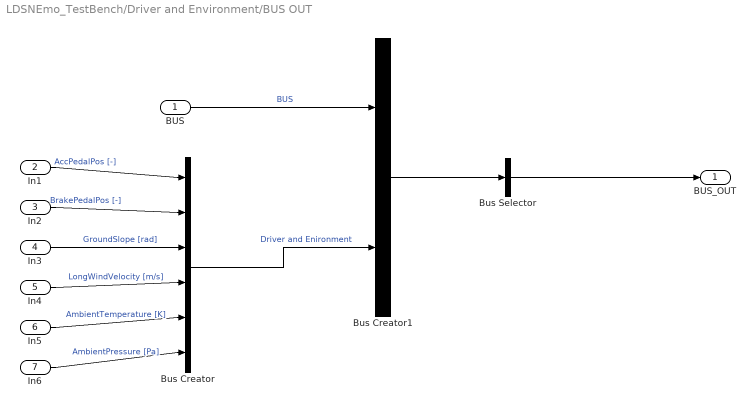
== system LDSNEmo_TestBench/Driver and Environment/BUS OUT ==
  BUS : Inport
  In1 : Inport  Port=2
  In2 : Inport  Port=3
  In3 : Inport  Port=4
  In4 : Inport  Port=5
  In5 : Inport  Port=6
  In6 : Inport  Port=7
  Bus Creator : BusCreator  Inputs=6
  Bus Creator1 : BusCreator  Inputs=2
  Bus Selector : BusSelector  OutputSignals=Driver and Enironment,BUS.DrivinCycle,BUS.Bus_Old  OutputAsBus=on
  BUS_OUT : Outport  VectorParamsAs1DForOutWhenUnconnected=off
  wires:
  Bus Creator1/1 -> Bus Selector/1
  BUS/1 -> Bus Creator1/1  "BUS"
  Bus Creator/1 -> Bus Creator1/2  "Driver and Enironment"
  Bus Selector/1 -> BUS_OUT/1
  In1/1 -> Bus Creator/1  "AccPedalPos [-]"
  In2/1 -> Bus Creator/2  "BrakePedalPos [-]"
  In3/1 -> Bus Creator/3  "GroundSlope [rad]"
  In4/1 -> Bus Creator/4  "LongWindVelocity [m/s]"
  In5/1 -> Bus Creator/5  "AmbientTemperature [K]"
  In6/1 -> Bus Creator/6  "AmbientPressure [Pa]"

== system LDSNEmo_TestBench/Driving Cycle/BUS IN ==
  BUS_In : Inport
  Bus Selector : BusSelector  OutputSignals=Bus_Old.Dynamics.VehSpd [m/s]
  BUS : Outport  VectorParamsAs1DForOutWhenUnconnected=off
  VehSpd [m/s] : Outport  Port=2  VectorParamsAs1DForOutWhenUnconnected=off
  wires:
  BUS_In/1 -> Bus Selector/1, BUS/1
  Bus Selector/1 -> VehSpd [m/s]/1  "<VehSpd [m/s]>"

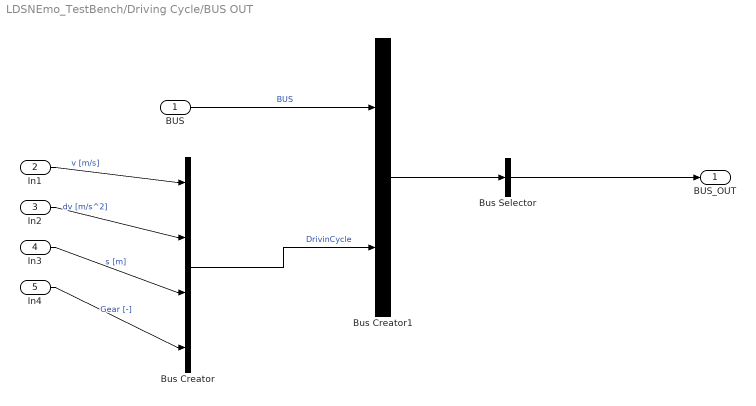
== system LDSNEmo_TestBench/Driving Cycle/BUS OUT ==
  BUS : Inport
  In1 : Inport  Port=2
  In2 : Inport  Port=3
  In3 : Inport  Port=4
  In4 : Inport  Port=5
  Bus Creator : BusCreator  Inputs=4
  Bus Creator1 : BusCreator  Inputs=2
  Bus Selector : BusSelector  OutputSignals=DrivinCycle,BUS.Bus_Old  OutputAsBus=on
  BUS_OUT : Outport  VectorParamsAs1DForOutWhenUnconnected=off
  wires:
  Bus Creator1/1 -> Bus Selector/1
  BUS/1 -> Bus Creator1/1  "BUS"
  Bus Creator/1 -> Bus Creator1/2  "DrivinCycle"
  Bus Selector/1 -> BUS_OUT/1
  In1/1 -> Bus Creator/1  "v [m/s]"
  In2/1 -> Bus Creator/2  "dv [m/s^2]"
  In3/1 -> Bus Creator/3  "s [m]"
  In4/1 -> Bus Creator/4  "Gear [-]"

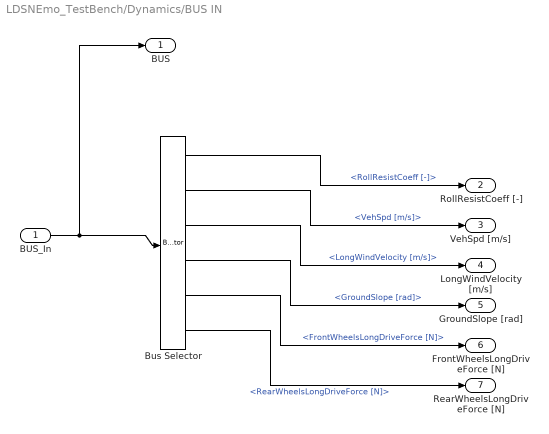
== system LDSNEmo_TestBench/Dynamics/BUS IN ==
  BUS_In : Inport
  Bus Selector : BusSelector  OutputSignals=Powertrain.RollResistCoeff [-],Bus_Old.Dynamics.VehSpd [m/s],Driver and Enironment.LongWindVelocity [m/s],Driver and Enironment.GroundSlope [rad],Powertrain.FrontWheelsLongDriveForce [N],Powertrain.RearWheelsLongDriveForce [N]
  BUS : Outport  VectorParamsAs1DForOutWhenUnconnected=off
  RollResistCoeff [-] : Outport  Port=2  VectorParamsAs1DForOutWhenUnconnected=off
  VehSpd [m/s] : Outport  Port=3  VectorParamsAs1DForOutWhenUnconnected=off
  LongWindVelocity [m/s] : Outport  Port=4  VectorParamsAs1DForOutWhenUnconnected=off
  GroundSlope [rad] : Outport  Port=5  VectorParamsAs1DForOutWhenUnconnected=off
  FrontWheelsLongDriveForce [N] : Outport  Port=6  VectorParamsAs1DForOutWhenUnconnected=off
  RearWheelsLongDriveForce [N] : Outport  Port=7  VectorParamsAs1DForOutWhenUnconnected=off
  wires:
  BUS_In/1 -> Bus Selector/1, BUS/1
  Bus Selector/1 -> RollResistCoeff [-]/1  "<RollResistCoeff [-]>"
  Bus Selector/2 -> VehSpd [m/s]/1  "<VehSpd [m/s]>"
  Bus Selector/3 -> LongWindVelocity [m/s]/1  "<LongWindVelocity [m/s]>"
  Bus Selector/4 -> GroundSlope [rad]/1  "<GroundSlope [rad]>"
  Bus Selector/5 -> FrontWheelsLongDriveForce [N]/1  "<FrontWheelsLongDriveForce [N]>"
  Bus Selector/6 -> RearWheelsLongDriveForce [N]/1  "<RearWheelsLongDriveForce [N]>"

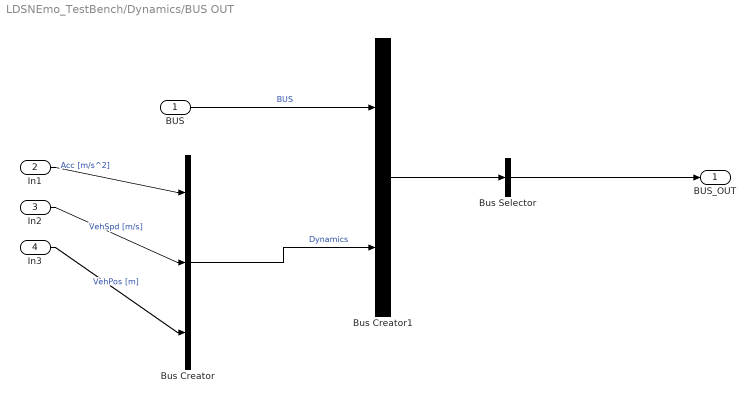
== system LDSNEmo_TestBench/Dynamics/BUS OUT ==
  BUS : Inport
  In1 : Inport  Port=2
  In2 : Inport  Port=3
  In3 : Inport  Port=4
  Bus Creator : BusCreator  Inputs=3
  Bus Creator1 : BusCreator  Inputs=2
  Bus Selector : BusSelector  OutputSignals=Dynamics,BUS.Powertrain,BUS.Powersource,BUS.VehicleControlUnit,BUS.Driver and Enironment,BUS.DrivinCycle,BUS.Bus_Old  OutputAsBus=on
  BUS_OUT : Outport  VectorParamsAs1DForOutWhenUnconnected=off
  wires:
  Bus Creator1/1 -> Bus Selector/1
  BUS/1 -> Bus Creator1/1  "BUS"
  Bus Creator/1 -> Bus Creator1/2  "Dynamics"
  Bus Selector/1 -> BUS_OUT/1
  In1/1 -> Bus Creator/1  "Acc [m/s^2]"
  In2/1 -> Bus Creator/2  "VehSpd [m/s]"
  In3/1 -> Bus Creator/3  "VehPos [m]"

== system LDSNEmo_TestBench/Power Source/BUS IN ==
  BUS_In : Inport
  Bus Selector : BusSelector  OutputSignals=Bus_Old.Powertrain.PowertrainPowerReq [W]
  BUS : Outport  VectorParamsAs1DForOutWhenUnconnected=off
  PowertrainPowerReq [W] : Outport  Port=2  VectorParamsAs1DForOutWhenUnconnected=off
  wires:
  BUS_In/1 -> Bus Selector/1, BUS/1
  Bus Selector/1 -> PowertrainPowerReq [W]/1  "<PowertrainPowerReq [W]>"

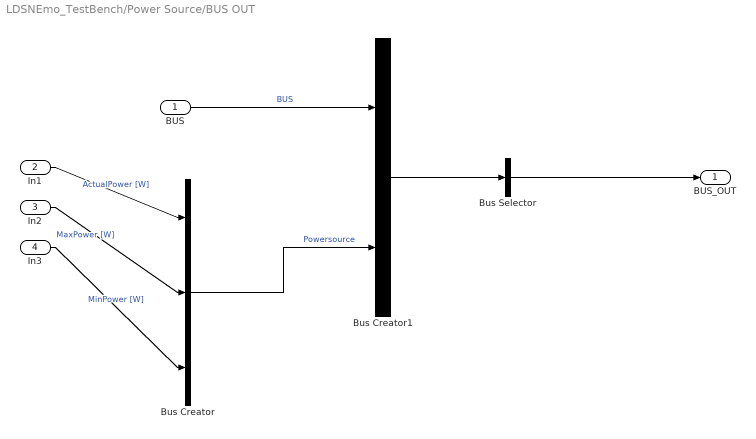
== system LDSNEmo_TestBench/Power Source/BUS OUT ==
  BUS : Inport
  In1 : Inport  Port=2
  In2 : Inport  Port=3
  In3 : Inport  Port=4
  Bus Creator : BusCreator  Inputs=3
  Bus Creator1 : BusCreator  Inputs=2
  Bus Selector : BusSelector  OutputSignals=Powersource,BUS.VehicleControlUnit,BUS.Driver and Enironment,BUS.DrivinCycle,BUS.Bus_Old  OutputAsBus=on
  BUS_OUT : Outport  VectorParamsAs1DForOutWhenUnconnected=off
  wires:
  Bus Creator1/1 -> Bus Selector/1
  BUS/1 -> Bus Creator1/1  "BUS"
  Bus Creator/1 -> Bus Creator1/2  "Powersource"
  Bus Selector/1 -> BUS_OUT/1
  In1/1 -> Bus Creator/1  "ActualPower [W]"
  In2/1 -> Bus Creator/2  "MaxPower [W]"
  In3/1 -> Bus Creator/3  "MinPower [W]"

== system LDSNEmo_TestBench/Power Source/Constant Power Source ==
  RequiredPower [W] : Inport
  Constant : Constant  Value=MaxPower
  Constant1 : Constant  Value=MinPower
  Saturation : Saturate  UpperLimit=MaxPower  LowerLimit=MinPower
  ActualPower [W] : Outport  VectorParamsAs1DForOutWhenUnconnected=off
  MaxPower [W] : Outport  Port=2  VectorParamsAs1DForOutWhenUnconnected=off
  MinPower [W] : Outport  Port=3  VectorParamsAs1DForOutWhenUnconnected=off
  wires:
  Constant/1 -> MaxPower [W]/1
  Constant1/1 -> MinPower [W]/1
  Saturation/1 -> ActualPower [W]/1
  RequiredPower [W]/1 -> Saturation/1

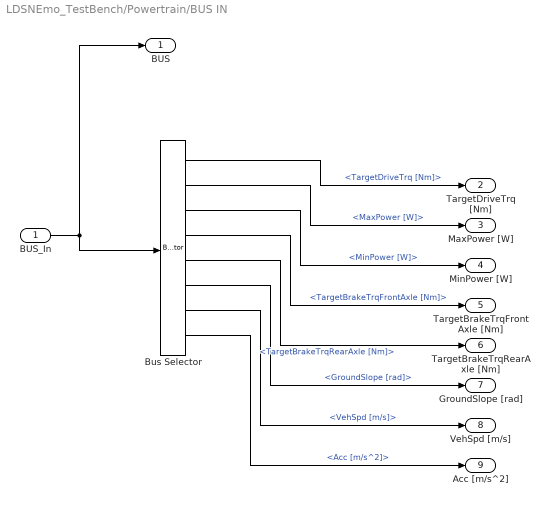
== system LDSNEmo_TestBench/Powertrain/BUS IN ==
  BUS_In : Inport
  Bus Selector : BusSelector  OutputSignals=VehicleControlUnit.TargetDriveTrq [Nm],Powersource.MaxPower [W],Powersource.MinPower [W],VehicleControlUnit.TargetBrakeTrqFrontAxle [Nm],VehicleControlUnit.TargetBrakeTrqRearAxle [Nm],Driver and Enironment.GroundSlope [rad],Bus_Old.Dynamics.VehSpd [m/s],Bus_Old.Dynamics.Acc [m/s^2]
  BUS : Outport  VectorParamsAs1DForOutWhenUnconnected=off
  TargetDriveTrq [Nm] : Outport  Port=2  VectorParamsAs1DForOutWhenUnconnected=off
  MaxPower [W] : Outport  Port=3  VectorParamsAs1DForOutWhenUnconnected=off
  MinPower [W] : Outport  Port=4  VectorParamsAs1DForOutWhenUnconnected=off
  TargetBrakeTrqFrontAxle [Nm] : Outport  Port=5  VectorParamsAs1DForOutWhenUnconnected=off
  TargetBrakeTrqRearAxle [Nm] : Outport  Port=6  VectorParamsAs1DForOutWhenUnconnected=off
  GroundSlope [rad] : Outport  Port=7  VectorParamsAs1DForOutWhenUnconnected=off
  VehSpd [m/s] : Outport  Port=8  VectorParamsAs1DForOutWhenUnconnected=off
  Acc [m/s^2] : Outport  Port=9  VectorParamsAs1DForOutWhenUnconnected=off
  wires:
  BUS_In/1 -> Bus Selector/1, BUS/1
  Bus Selector/1 -> TargetDriveTrq [Nm]/1  "<TargetDriveTrq [Nm]>"
  Bus Selector/2 -> MaxPower [W]/1  "<MaxPower [W]>"
  Bus Selector/3 -> MinPower [W]/1  "<MinPower [W]>"
  Bus Selector/4 -> TargetBrakeTrqFrontAxle [Nm]/1  "<TargetBrakeTrqFrontAxle [Nm]>"
  Bus Selector/5 -> TargetBrakeTrqRearAxle [Nm]/1  "<TargetBrakeTrqRearAxle [Nm]>"
  Bus Selector/6 -> GroundSlope [rad]/1  "<GroundSlope [rad]>"
  Bus Selector/7 -> VehSpd [m/s]/1  "<VehSpd [m/s]>"
  Bus Selector/8 -> Acc [m/s^2]/1  "<Acc [m/s^2]>"

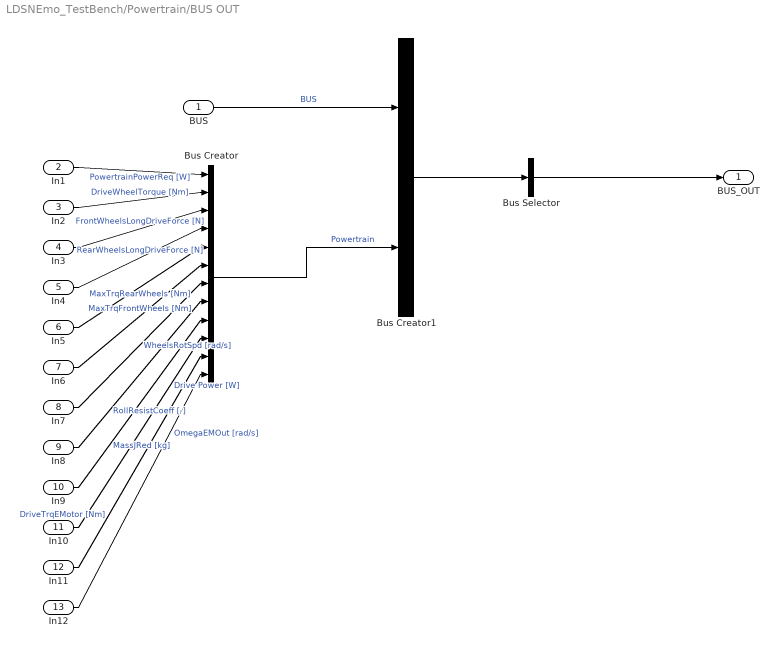
== system LDSNEmo_TestBench/Powertrain/BUS OUT ==
  BUS : Inport
  In1 : Inport  Port=2
  In2 : Inport  Port=3
  In3 : Inport  Port=4
  In4 : Inport  Port=5
  In5 : Inport  Port=6
  In6 : Inport  Port=7
  In7 : Inport  Port=8
  In8 : Inport  Port=9
  In9 : Inport  Port=10
  In10 : Inport  Port=11
  In11 : Inport  Port=12
  In12 : Inport  Port=13
  Bus Creator : BusCreator  Inputs=12
  Bus Creator1 : BusCreator  Inputs=2
  Bus Selector : BusSelector  OutputSignals=Powertrain,BUS.Powersource,BUS.VehicleControlUnit,BUS.Driver and Enironment,BUS.DrivinCycle,BUS.Bus_Old  OutputAsBus=on
  BUS_OUT : Outport  VectorParamsAs1DForOutWhenUnconnected=off
  wires:
  Bus Creator1/1 -> Bus Selector/1
  BUS/1 -> Bus Creator1/1  "BUS"
  Bus Creator/1 -> Bus Creator1/2  "Powertrain"
  Bus Selector/1 -> BUS_OUT/1
  In1/1 -> Bus Creator/1  "PowertrainPowerReq [W]"
  In2/1 -> Bus Creator/2  "DriveWheelTorque [Nm]"
  In3/1 -> Bus Creator/3  "FrontWheelsLongDriveForce [N]"
  In4/1 -> Bus Creator/4  "RearWheelsLongDriveForce [N]"
  In5/1 -> Bus Creator/5  "MaxTrqRearWheels [Nm]"
  In6/1 -> Bus Creator/6  "MaxTrqFrontWheels [Nm]"
  In7/1 -> Bus Creator/7  "WheelsRotSpd [rad/s]"
  In8/1 -> Bus Creator/8  "RollResistCoeff [-]"
  In9/1 -> Bus Creator/9  "MassJRed [kg]"
  In10/1 -> Bus Creator/10  "Drive Power [W]"
  In11/1 -> Bus Creator/11  "DriveTrqEMotor [Nm]"
  In12/1 -> Bus Creator/12  "OmegaEMOut [rad/s]"
